simulink model "sf_aircontrol_exercise"  (R2015a)
settings: Solver=ode45  StartTime=0.0  StopTime=600  FixedStep=1000  RelTol=1e-3
undefined symbols (not defined in the file): sigbuilder_block
settings Model: CovSFcnEnable=off  ExtModeAutoUpdateStatusClock=off  Creator=The MathWorks, Inc.  LastModifiedBy=ktrinh
settings SolverCC: MaxConsecutiveZCs=500
settings OptimizationCC: ExpressionDepthLimit=2147483647  InitFltsAndDblsToZero=on
settings DebuggingCC: UnderspecifiedInitializationDetection=Classic  MergeDetectMultiDrivingBlocksExec=none  SignalResolutionControl=TryResolveAllWithWarning  MultiTaskDSMMsg=warning  MultiTaskCondExecSysMsg=none  FcnCallInpInsideContextMsg=EnableAllAsWarning  StateNameClashWarn=warning  StrictBusMsg=Warning
settings GRTTargetCC: TargetFcnLib=ansi_tfl_tmw.mat  CombineOutputUpdateFcns=off  GRTInterface=on

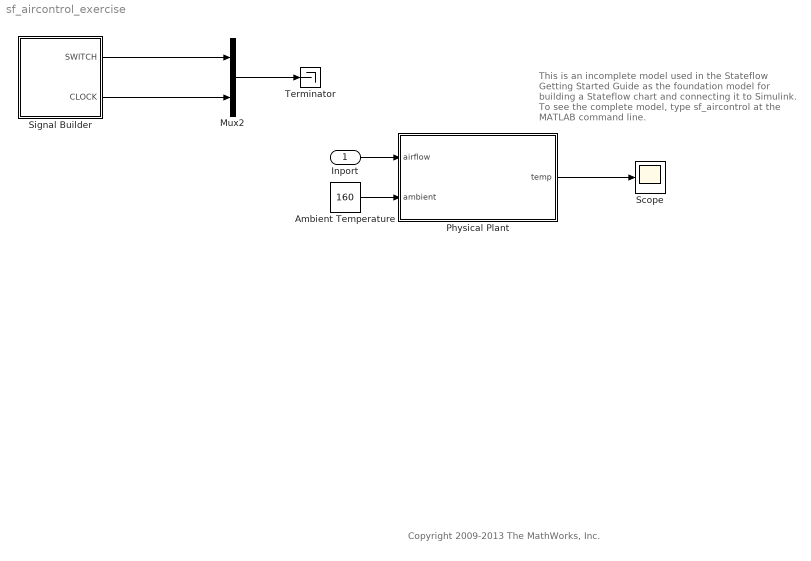
== system sf_aircontrol_exercise ==
  note: This is an incomplete model
      | used in the Stateflow Getting Started Guide
      | as the foundation model for building
      |  a Stateflow chart and connecting it to Simulink.
      | To see the complete model, type sf_aircontrol
      | at the MATLAB command line.
  note: Copyright 2009-2013 The MathWorks, Inc.
  Inport : Inport
  Ambient Temperature : Constant  Value=160
  Mux2 : Mux  Inputs=2
  Physical Plant : Subsystem
  Scope : Scope
      settings: TimeRange=600  MaxDataPoints=5000  SaveToWorkspace=off  SaveName=ScopeData  YMin=60  YMax=160  SampleTime=-1
  Signal Builder : Subsystem  Tag=STV Subsys  LoadFcn=sigbuilder_block('load');  StartFcn=sigbuilder_block('start');  StopFcn=sigbuilder_block('stop');  ClipboardFcn=sigbuilder_block('clipboard');  mask(Sigbuilder block){}
      mask help: Sigbuilder GUI
      mask init:
      | if ~strcmp(get_param(bdroot(gcbh),'SimulationStatus'),'stopped') tuvar = sigbuilder_block('maskInit'); end
      settings: CopyFcn=sigbuilder_block('copy');  DeleteFcn=sigbuilder_block('delete');  ModelCloseFcn=sigbuilder_block('modelClose');  PreSaveFcn=sigbuilder_block('preSave');  PauseFcn=sigbuilder_block('pause')  ContinueFcn=sigbuilder_block('continue')  NameChangeFcn=sigbuilder_block('namechange');  OpenFcn=sigbuilder_block('open',[88.5 78 603 348.75 ]);  CloseFcn=sigbuilder_block('close');
      mask Display: plot(0, 0, 100, 100,[2, 2, 32, 32, 2], [68, 8, 8, 68, 68],[32, 2], [38, 38], [32, 19, 2],[53, 60, 44], [32, 17, 17, 2],[16, 16, 31, 31]);txt = getActiveGroup(gcbh);text(2, 100, txt,'verticalAlignment', 'top');
  Terminator : Terminator
  wires:
  Ambient Temperature/1 -> Physical Plant/2(ambient)
  Physical Plant/1(temp) -> Scope/1
  Signal Builder/1(SWITCH) -> Mux2/1
  Signal Builder/2(CLOCK) -> Mux2/2
  Mux2/1 -> Terminator/1
  Inport/1 -> Physical Plant/1(airflow)

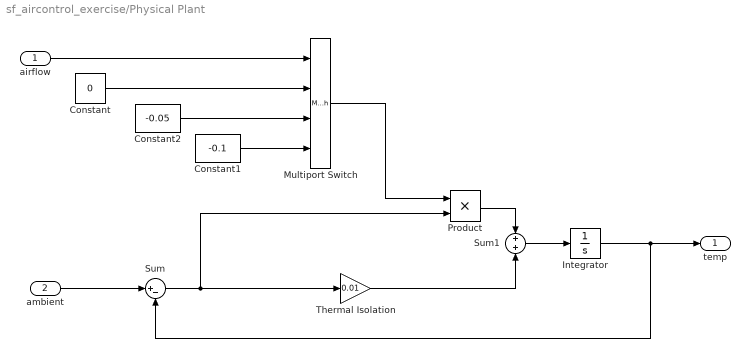
== system sf_aircontrol_exercise/Physical Plant ==
  airflow : Inport
  ambient : Inport  Port=2
  Constant : Constant  Value=0
  Constant1 : Constant  Value=-0.1
  Constant2 : Constant  Value=-0.05
  Integrator : Integrator  InitialCondition=70
  Multiport Switch : MultiPortSwitch  DataPortOrder=Zero-based contiguous  zeroidx=on
  Product : Product  RndMeth=Zero
  Sum : Sum  Inputs=|+-
  Sum1 : Sum  Inputs=+|+
  Thermal Isolation : Gain  Gain=0.01
  temp : Outport
  wires:
  Integrator/1 -> temp/1, Sum/2
  Sum1/1 -> Integrator/1
  Constant2/1 -> Multiport Switch/3
  Constant/1 -> Multiport Switch/2
  airflow/1 -> Multiport Switch/1
  ambient/1 -> Sum/1
  Sum/1 -> Thermal Isolation/1, Product/2
  Product/1 -> Sum1/1
  Thermal Isolation/1 -> Sum1/2
  Multiport Switch/1 -> Product/1
  Constant1/1 -> Multiport Switch/4

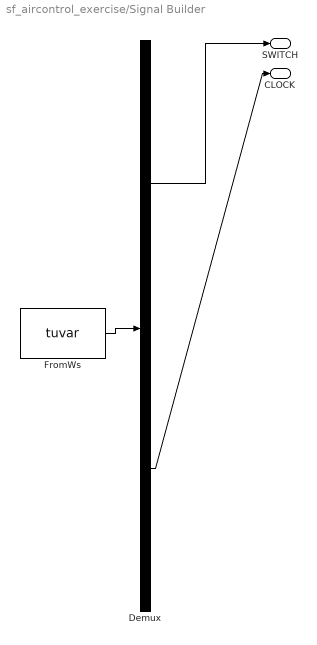
== system sf_aircontrol_exercise/Signal Builder ==
  Demux : Demux  Tag=STV Demux  Outputs=2
  FromWs : FromWorkspace  Tag=STV FromWs  VariableName=tuvar  SampleTime=0
      SigBuilderData=|
      | common.afterFinalStr = 'Extrapolate'
      | common.sampleTime = 0
      | dataSet.timeRange = [0 600]
      | dataSet.name = 'Group 1'
      | sbobj.Groups.Name = 'Group 1'
      | sbobj.Groups.Signals(1).Name = 'SWITCH'
      | sbobj.Groups.Signals(1).XData = [0 350 350 501 501 600]
      | sbobj.Groups.Signals(1).YData = [0 -0.01 1 1 0 0]
      | sbobj.Groups.Signals(2).Name = 'CLOCK'
      | sbobj.Groups.Signals(2).XData = [0 0.5 0.5 1 1 1.5 1.5 2 2 2.5 2.5 3 ... (2397 elements, 1x2397)]
      | sbobj.Groups.Signals(2).YData = [2 2 0 0 2 2 0 0 2 2 0 0 ... (2397 elements, 1x2397)]
      | sbobj.Groups.TimeRange = [0 600]
  SWITCH : Outport  Tag=STV Outport
  CLOCK : Outport  Tag=STV Outport  Port=2
  wires:
  Demux/1 -> SWITCH/1
  FromWs/1 -> Demux/1
  Demux/2 -> CLOCK/1
